simulink model "Logging"  (Simulink 9.1)
settings: Solver=VariableStepAuto  StartTime=0.0  StopTime=10.0  RelTol=1e-3
settings Model: LogicAnalyzerSignalOrdering=8bf68fb7-e9c2-472a-a2d5-0b6182d7556c  Creator=dongw  LastModifiedBy=dongw
settings DataIOCC: SaveFormat=Dataset
settings OptimizationCC: LifeSpan=auto
settings DebuggingCC: UnderspecifiedInitializationDetection=Simplified  MergeDetectMultiDrivingBlocksExec=error  SFUnexpectedBacktrackingDiag=error  SFNoUnconditionalDefaultTransitionDiag=error  SFExecutionAtInitializationDiag=warning
settings HardwareCC: ProdBitPerPointer=64  ProdBitPerSizeT=64  ProdBitPerPtrDiffT=64  ProdLargestAtomicFloat=Float  ProdIntDivRoundTo=Zero  ProdEndianess=LittleEndian  ProdWordSize=64  ProdHWDeviceType=Intel->x86-64 (Windows64)
settings ModelReferenceCC: PropagateSignalLabelsOutOfModel=on
settings CodeAppCC: StateflowObjectComments=off
settings GRTTargetCC: TargetLangStandard=C99 (ISO)  CombineOutputUpdateFcns=on  GRTInterface=off
settings ConfigComp: CovMetricSettings=dwe  CovHtmlReporting=off  CovSaveCumulativeToWorkspaceVar=off  CovSaveSingleToWorkspaceVar=off  CovExternalEMLEnable=on

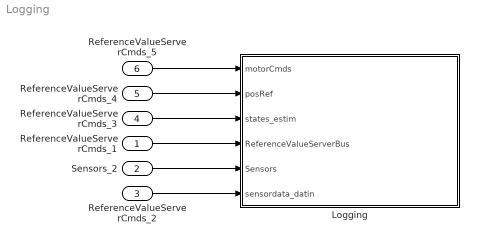
== system Logging ==
  ReferenceValueServerCmds_1 : Inport  OutDataTypeStr=Bus: CommandBus
  Sensors_2 : Inport  Port=2  OutDataTypeStr=Bus: SensorsBus  BusOutputAsStruct=on
  ReferenceValueServerCmds_2 : Inport  Port=3  OutDataTypeStr=Bus: CommandBus
  ReferenceValueServerCmds_3 : Inport  Port=4  OutDataTypeStr=Bus: CommandBus
  ReferenceValueServerCmds_4 : Inport  Port=5  OutDataTypeStr=Bus: CommandBus
  ReferenceValueServerCmds_5 : Inport  Port=6  OutDataTypeStr=Bus: CommandBus
  Logging : Subsystem  TreatAsAtomicUnit=on
      settings: RTWFcnNameOpts=Use subsystem name
  wires:
  ReferenceValueServerCmds_4/1 -> Logging/2(posRef)
  ReferenceValueServerCmds_3/1 -> Logging/3(states_estim)
  Sensors_2/1 -> Logging/5(Sensors)
  ReferenceValueServerCmds_1/1 -> Logging/4(ReferenceValueServerBus)
  ReferenceValueServerCmds_2/1 -> Logging/6(sensordata_datin)
  ReferenceValueServerCmds_5/1 -> Logging/1(motorCmds)

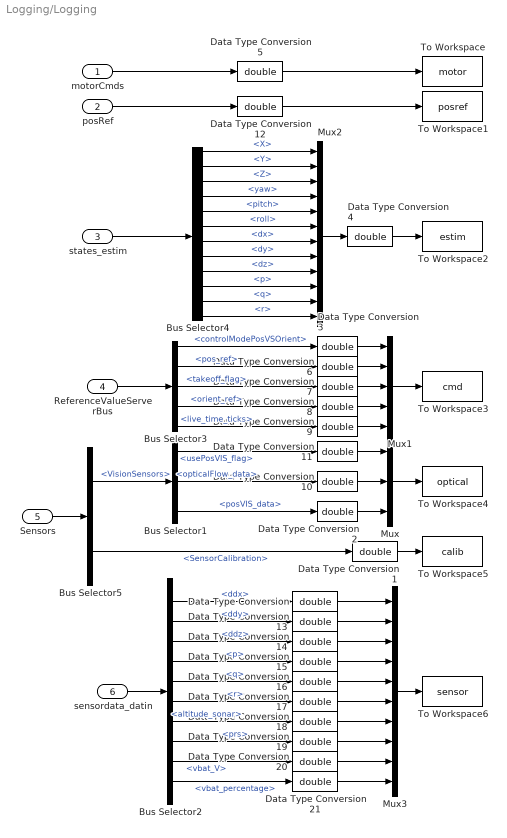
== system Logging/Logging ==
  motorCmds : Inport
  posRef : Inport  Port=2
  states_estim : Inport  Port=3  OutDataTypeStr=Bus: statesEstim_t  BusOutputAsStruct=on
  ReferenceValueServerBus : Inport  Port=4  OutDataTypeStr=Bus: CommandBus  BusOutputAsStruct=on
  Sensors : Inport  Port=5  OutDataTypeStr=Bus: SensorsBus
  sensordata_datin : Inport  Port=6  OutDataTypeStr=Bus: sensordata_t
  Bus Selector1 : BusSelector  OutputSignals=usePosVIS_flag,opticalFlow_data,posVIS_data
  Bus Selector2 : BusSelector  OutputSignals=ddx,ddy,ddz,p,q,r,altitude_sonar,prs,vbat_V,vbat_percentage
  Bus Selector3 : BusSelector  OutputSignals=controlModePosVSOrient,pos_ref,takeoff_flag,orient_ref,live_time_ticks
  Bus Selector4 : BusSelector  OutputSignals=X,Y,Z,yaw,pitch,roll,dx,dy,dz,p,q,r
  Bus Selector5 : BusSelector  OutputSignals=VisionSensors,SensorCalibration
  Data Type Conversion{,1..21} (22 alike) : DataTypeConversion  OutDataTypeStr=double
  Mux : Mux  Inputs=3
  Mux1 : Mux  Inputs=5
  Mux2 : Mux  Inputs=12
  Mux3 : Mux  Inputs=10
  To Workspace : ToWorkspace  VariableName=motor  SaveFormat=Structure With Time  SampleTime=-1
  To Workspace1 : ToWorkspace  VariableName=posref  SaveFormat=Structure With Time  SampleTime=-1
  To Workspace2 : ToWorkspace  VariableName=estim  SaveFormat=Structure With Time  SampleTime=-1
  To Workspace3 : ToWorkspace  VariableName=cmd  SaveFormat=Structure With Time  SampleTime=-1
  To Workspace4 : ToWorkspace  VariableName=optical  SaveFormat=Structure With Time  SampleTime=-1
  To Workspace5 : ToWorkspace  VariableName=calib  SaveFormat=Structure With Time  SampleTime=-1
  To Workspace6 : ToWorkspace  VariableName=sensor  SaveFormat=Structure With Time  SampleTime=-1
  wires:
  Bus Selector3/1 -> Data Type Conversion3/1  "<controlModePosVSOrient>"
  Bus Selector3/3 -> Data Type Conversion7/1  "<takeoff_flag>"
  Bus Selector3/4 -> Data Type Conversion8/1  "<orient_ref>"
  Bus Selector3/5 -> Data Type Conversion9/1  "<live_time_ticks>"
  ReferenceValueServerBus/1 -> Bus Selector3/1
  Bus Selector3/2 -> Data Type Conversion6/1  "<pos_ref>"
  sensordata_datin/1 -> Bus Selector2/1
  Bus Selector2/1 -> Data Type Conversion/1  "<ddx>"
  Sensors/1 -> Bus Selector5/1
  Bus Selector1/1 -> Data Type Conversion11/1  "<usePosVIS_flag>"
  Bus Selector1/2 -> Data Type Conversion10/1  "<opticalFlow_data>"
  Bus Selector1/3 -> Data Type Conversion2/1  "<posVIS_data>"
  Data Type Conversion1/1 -> To Workspace5/1
  Bus Selector5/2 -> Data Type Conversion1/1  "<SensorCalibration>"
  Mux/1 -> To Workspace4/1
  Data Type Conversion4/1 -> To Workspace2/1
  motorCmds/1 -> Data Type Conversion5/1
  Data Type Conversion5/1 -> To Workspace/1
  Mux1/1 -> To Workspace3/1
  states_estim/1 -> Bus Selector4/1
  Mux2/1 -> Data Type Conversion4/1
  Bus Selector4/4 -> Mux2/4  "<yaw>"
  Bus Selector4/6 -> Mux2/6  "<roll>"
  Bus Selector4/5 -> Mux2/5  "<pitch>"
  Bus Selector4/9 -> Mux2/9  "<dz>"
  Bus Selector4/7 -> Mux2/7  "<dx>"
  Bus Selector4/8 -> Mux2/8  "<dy>"
  Bus Selector4/10 -> Mux2/10  "<p>"
  Bus Selector4/12 -> Mux2/12  "<r>"
  Bus Selector4/2 -> Mux2/2  "<Y>"
  Bus Selector4/11 -> Mux2/11  "<q>"
  Bus Selector4/3 -> Mux2/3  "<Z>"
  Bus Selector4/1 -> Mux2/1  "<X>"
  Data Type Conversion3/1 -> Mux1/1
  Data Type Conversion6/1 -> Mux1/2
  Data Type Conversion7/1 -> Mux1/3
  Data Type Conversion8/1 -> Mux1/4
  Data Type Conversion9/1 -> Mux1/5
  Data Type Conversion2/1 -> Mux/3
  Data Type Conversion10/1 -> Mux/2
  Data Type Conversion11/1 -> Mux/1
  posRef/1 -> Data Type Conversion12/1
  Data Type Conversion12/1 -> To Workspace1/1
  Bus Selector2/2 -> Data Type Conversion13/1  "<ddy>"
  Bus Selector2/3 -> Data Type Conversion14/1  "<ddz>"
  Bus Selector2/4 -> Data Type Conversion15/1  "<p>"
  Bus Selector2/5 -> Data Type Conversion16/1  "<q>"
  Bus Selector2/6 -> Data Type Conversion17/1  "<r>"
  Bus Selector2/7 -> Data Type Conversion18/1  "<altitude_sonar>"
  Bus Selector2/8 -> Data Type Conversion19/1  "<prs>"
  Bus Selector2/9 -> Data Type Conversion20/1  "<vbat_V>"
  Bus Selector2/10 -> Data Type Conversion21/1  "<vbat_percentage>"
  Data Type Conversion/1 -> Mux3/1
  Data Type Conversion13/1 -> Mux3/2
  Data Type Conversion14/1 -> Mux3/3
  Data Type Conversion15/1 -> Mux3/4
  Data Type Conversion16/1 -> Mux3/5
  Data Type Conversion17/1 -> Mux3/6
  Data Type Conversion18/1 -> Mux3/7
  Data Type Conversion19/1 -> Mux3/8
  Data Type Conversion20/1 -> Mux3/9
  Data Type Conversion21/1 -> Mux3/10
  Mux3/1 -> To Workspace6/1
  Bus Selector5/1 -> Bus Selector1/1  "<VisionSensors>"
